simulink model "DC_MOTOR_differ_representation"  (R2015a)
settings: Solver=ode45  StartTime=0.0  StopTime=10.0  RelTol=1e-3
InitFcn:
  | clear
  | clc
  | 
  | 
  | 
  | Ke  =   0.57;
  | R    =  9.375
  | L    =   6e-4
  | Kt   =  0.2;
  | b    =  9.3e-3
  | J     =  5.26e-5
  | 
  | 
  | theta_dot0 = 0;
  | i0 = 0;
libraries: simulink x3
settings Model: Creator=Alfa maSR  LastModifiedBy=Alfa maSR

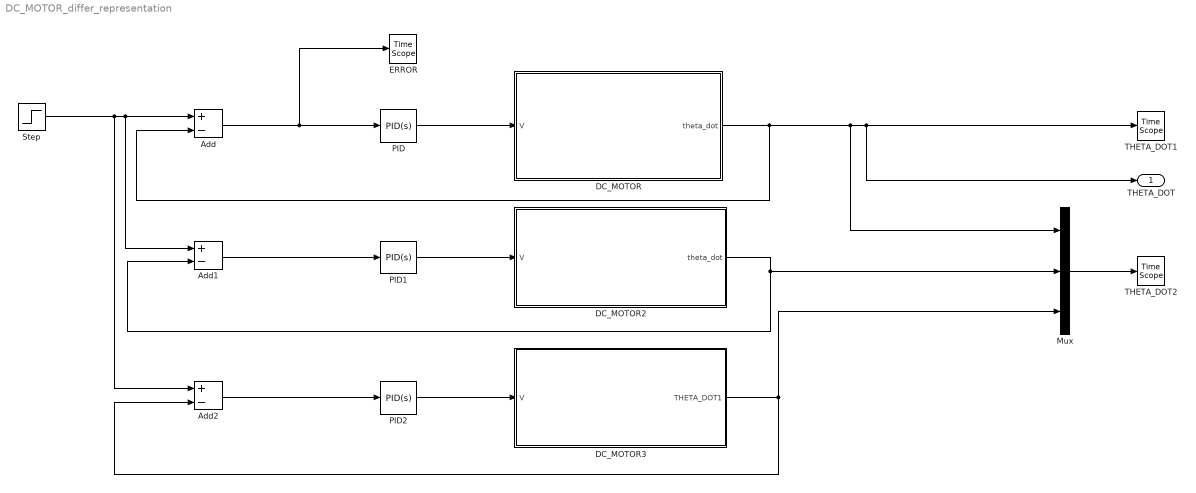
== system DC_MOTOR_differ_representation ==
  Add : Sum  Inputs=+-
  Add1 : Sum  Inputs=+-
  Add2 : Sum  Inputs=+-
  DC_MOTOR : Subsystem
  DC_MOTOR2 : Subsystem
  "DC_MOTOR3 " : Subsystem
  ERROR : TimeScope  DefaultConfigurationName=spbscopes.TimeScopeBlockCfg
  Mux : Mux  Inputs=3
  "PID " : simulink/Continuous/PID Controller  Controller=PID  TimeDomain=Continuous-time  SampleTime=-1  IntegratorMethod=Forward Euler  FilterMethod=Forward Euler  Form=Parallel  UseFilter=on  ControllerParametersSource=internal  P=1  I=1  D=0  N=100  InitialConditionSource=internal  InitialConditionForIntegrator=0  InitialConditionForFilter=0  ExternalReset=none  LimitOutput=off  UpperSaturationLimit=inf  LowerSaturationLimit=-inf  LinearizeAsGain=on  AntiWindupMode=none  Kb=1  TrackingMode=off  Kt=1  PParamMin=[]  PParamMax=[]  IParamMin=[]  IParamMax=[]  DParamMin=[]  DParamMax=[]  NParamMin=[]  NParamMax=[]  KbParamMin=[]  KbParamMax=[]  KtParamMin=[]  KtParamMax=[]  POutMin=[]  POutMax=[]  IOutMin=[]  IOutMax=[]  DOutMin=[]  DOutMax=[]  NOutMin=[]  NOutMax=[]  KbOutMin=[]  KbOutMax=[]  KtOutMin=[]  KtOutMax=[]  IntegratorOutMin=[]  IntegratorOutMax=[]  FilterOutMin=[]  FilterOutMax=[]  SumOutMin=[]  SumOutMax=[]  SumI1OutMin=[]  SumI1OutMax=[]  SumI2OutMin=[]  SumI2OutMax=[]  SumI3OutMin=[]  SumI3OutMax=[]  SumDOutMin=[]  SumDOutMax=[]  SaturationOutMin=[]  SaturationOutMax=[]  IntegratorContinuousStateAttributes=''  IntegratorStateMustResolveToSignalObject=off  IntegratorRTWStateStorageClass=Auto  FilterContinuousStateAttributes=''  FilterStateMustResolveToSignalObject=off  FilterRTWStateStorageClass=Auto  DifferentiatorICPrevScaledInput=0  DifferentiatorOutMin=[]  DifferentiatorOutMax=[]
  PID1 : simulink/Continuous/PID Controller  Controller=PID  TimeDomain=Continuous-time  SampleTime=-1  IntegratorMethod=Forward Euler  FilterMethod=Forward Euler  Form=Parallel  UseFilter=on  ControllerParametersSource=internal  P=1  I=1  D=0  N=100  InitialConditionSource=internal  InitialConditionForIntegrator=0  InitialConditionForFilter=0  ExternalReset=none  LimitOutput=off  UpperSaturationLimit=inf  LowerSaturationLimit=-inf  LinearizeAsGain=on  AntiWindupMode=none  Kb=1  TrackingMode=off  Kt=1  PParamMin=[]  PParamMax=[]  IParamMin=[]  IParamMax=[]  DParamMin=[]  DParamMax=[]  NParamMin=[]  NParamMax=[]  KbParamMin=[]  KbParamMax=[]  KtParamMin=[]  KtParamMax=[]  POutMin=[]  POutMax=[]  IOutMin=[]  IOutMax=[]  DOutMin=[]  DOutMax=[]  NOutMin=[]  NOutMax=[]  KbOutMin=[]  KbOutMax=[]  KtOutMin=[]  KtOutMax=[]  IntegratorOutMin=[]  IntegratorOutMax=[]  FilterOutMin=[]  FilterOutMax=[]  SumOutMin=[]  SumOutMax=[]  SumI1OutMin=[]  SumI1OutMax=[]  SumI2OutMin=[]  SumI2OutMax=[]  SumI3OutMin=[]  SumI3OutMax=[]  SumDOutMin=[]  SumDOutMax=[]  SaturationOutMin=[]  SaturationOutMax=[]  IntegratorContinuousStateAttributes=''  IntegratorStateMustResolveToSignalObject=off  IntegratorRTWStateStorageClass=Auto  FilterContinuousStateAttributes=''  FilterStateMustResolveToSignalObject=off  FilterRTWStateStorageClass=Auto  DifferentiatorICPrevScaledInput=0  DifferentiatorOutMin=[]  DifferentiatorOutMax=[]
  PID2 : simulink/Continuous/PID Controller  Controller=PID  TimeDomain=Continuous-time  SampleTime=-1  IntegratorMethod=Forward Euler  FilterMethod=Forward Euler  Form=Parallel  UseFilter=on  ControllerParametersSource=internal  P=1  I=1  D=0  N=100  InitialConditionSource=internal  InitialConditionForIntegrator=0  InitialConditionForFilter=0  ExternalReset=none  LimitOutput=off  UpperSaturationLimit=inf  LowerSaturationLimit=-inf  LinearizeAsGain=on  AntiWindupMode=none  Kb=1  TrackingMode=off  Kt=1  PParamMin=[]  PParamMax=[]  IParamMin=[]  IParamMax=[]  DParamMin=[]  DParamMax=[]  NParamMin=[]  NParamMax=[]  KbParamMin=[]  KbParamMax=[]  KtParamMin=[]  KtParamMax=[]  POutMin=[]  POutMax=[]  IOutMin=[]  IOutMax=[]  DOutMin=[]  DOutMax=[]  NOutMin=[]  NOutMax=[]  KbOutMin=[]  KbOutMax=[]  KtOutMin=[]  KtOutMax=[]  IntegratorOutMin=[]  IntegratorOutMax=[]  FilterOutMin=[]  FilterOutMax=[]  SumOutMin=[]  SumOutMax=[]  SumI1OutMin=[]  SumI1OutMax=[]  SumI2OutMin=[]  SumI2OutMax=[]  SumI3OutMin=[]  SumI3OutMax=[]  SumDOutMin=[]  SumDOutMax=[]  SaturationOutMin=[]  SaturationOutMax=[]  IntegratorContinuousStateAttributes=''  IntegratorStateMustResolveToSignalObject=off  IntegratorRTWStateStorageClass=Auto  FilterContinuousStateAttributes=''  FilterStateMustResolveToSignalObject=off  FilterRTWStateStorageClass=Auto  DifferentiatorICPrevScaledInput=0  DifferentiatorOutMin=[]  DifferentiatorOutMax=[]
  Step : Step  Time=0  SampleTime=0
  THETA_DOT1 : TimeScope  DefaultConfigurationName=spbscopes.TimeScopeBlockCfg
  THETA_DOT2 : TimeScope  DefaultConfigurationName=spbscopes.TimeScopeBlockCfg
  THETA_DOT : Outport
  wires:
  DC_MOTOR/1(theta_dot) -> Add/2, THETA_DOT1/1, THETA_DOT/1, Mux/1
  "PID "/1 -> DC_MOTOR/1(V)
  Step/1 -> Add2/1, Add1/1, Add/1
  Add/1 -> ERROR/1, "PID "/1
  Add1/1 -> PID1/1
  PID1/1 -> DC_MOTOR2/1(V)
  DC_MOTOR2/1(theta_dot) -> Add1/2, Mux/2
  Add2/1 -> PID2/1
  PID2/1 -> "DC_MOTOR3 "/1(V)
  "DC_MOTOR3 "/1(THETA_DOT1) -> Mux/3, Add2/2
  Mux/1 -> THETA_DOT2/1

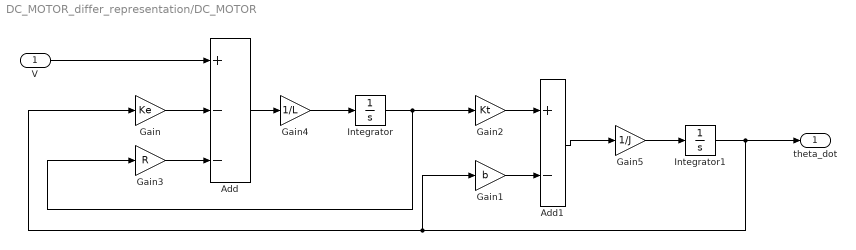
== system DC_MOTOR_differ_representation/DC_MOTOR ==
  V : Inport
  Add : Sum  Inputs=+--
  Add1 : Sum  Inputs=+-
  Gain : Gain  Gain=Ke
  Gain1 : Gain  Gain=b
  Gain2 : Gain  Gain=Kt
  Gain3 : Gain  Gain=R
  Gain4 : Gain  Gain=1/L
  Gain5 : Gain  Gain=1/J
  Integrator : Integrator  InitialCondition=i0
  Integrator1 : Integrator  InitialCondition=theta_dot0
  theta_dot : Outport
  wires:
  Add1/1 -> Gain5/1
  Gain1/1 -> Add1/2
  Integrator1/1 -> theta_dot/1, Gain/1, Gain1/1
  Add/1 -> Gain4/1
  Gain4/1 -> Integrator/1
  Gain2/1 -> Add1/1
  Integrator/1 -> Gain3/1, Gain2/1
  Gain3/1 -> Add/3
  Gain/1 -> Add/2
  V/1 -> Add/1
  Gain5/1 -> Integrator1/1

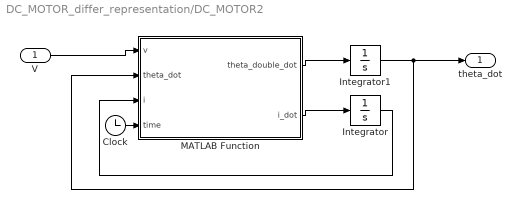
== system DC_MOTOR_differ_representation/DC_MOTOR2 ==
  V : Inport
  Clock : Clock
  Integrator : Integrator  InitialCondition=i0
  Integrator1 : Integrator  InitialCondition=theta_dot0
  MATLAB Function : MATLAB Function  TreatAsAtomicUnit=on
  theta_dot : Outport
  wires:
  Integrator/1 -> MATLAB Function/3(i)
  Integrator1/1 -> theta_dot/1, MATLAB Function/2(theta_dot)
  MATLAB Function/1(theta_double_dot) -> Integrator1/1
  MATLAB Function/2(i_dot) -> Integrator/1
  V/1 -> MATLAB Function/1(v)
  Clock/1 -> MATLAB Function/4(time)

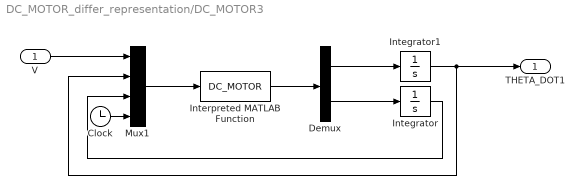
== system DC_MOTOR_differ_representation/DC_MOTOR3  ==
  V : Inport
  Clock : Clock
  Demux : Demux  Outputs=2
  Integrator : Integrator  InitialCondition=i0
  Integrator1 : Integrator  InitialCondition=theta_dot0
  Interpreted MATLAB Function : MATLABFcn  MATLABFcn=DC_MOTOR  OutputDimensions=2
  Mux1 : Mux
  THETA_DOT1 : Outport
  wires:
  Mux1/1 -> Interpreted MATLAB Function/1
  Demux/2 -> Integrator/1
  Integrator1/1 -> THETA_DOT1/1, Mux1/2
  Demux/1 -> Integrator1/1
  Interpreted MATLAB Function/1 -> Demux/1
  Integrator/1 -> Mux1/3
  V/1 -> Mux1/1
  Clock/1 -> Mux1/4

== matlab function DC_MOTOR_differ_representation/DC_MOTOR2/MATLAB Function ==
  data: v input; theta_double_dot output; theta_dot input; i input; i_dot output; time input
function [theta_double_dot,i_dot] = fcn(v , theta_dot, i ,time )

% motor characteristics ..

Ke = 0.57;           % electromotive force constant.
R  = 9.375 ;         % electric resistance.
L  = 6e-4;           % electric inductance.
Kt = 0.2;            % motor torque constant.
b  = 9.3e-3;         % motor ciscous friction constant. 
J  = 5.26e-5;        % moment of inertia of the rotor.


theta_double_dot = ( Kt*i - b* theta_dot)/J ;
i_dot = ( v- Ke*theta_dot - R*i)/L;
